simulink model "A13_17"  (R2017b)
settings: Solver=VariableStepAuto  StartTime=0.0  StopTime=20  RelTol=1e-3
settings Model: Creator=user  LastModifiedBy=user
settings SFSimCC: SimUseLocalCustomCode=on
settings RTWCC: RTWUseLocalCustomCode=on

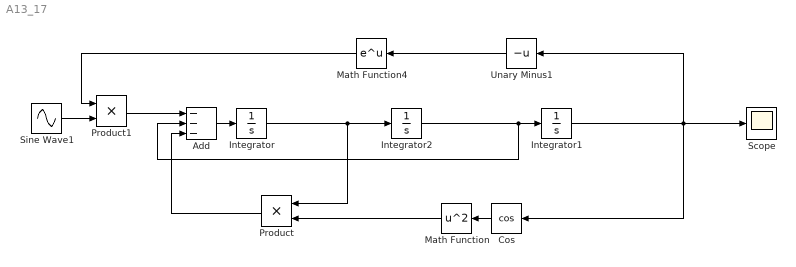
== system A13_17 ==
  Add : Sum  Inputs=---
  Cos : Trigonometry  Operator=cos
  Integrator : Integrator  InitialCondition=1
  Integrator1 : Integrator  InitialCondition=3
  Integrator2 : Integrator  InitialCondition=-2
  Math Function : Math  Operator=square  SaturateOnIntegerOverflow=on
  Math Function4 : Math  SaturateOnIntegerOverflow=on
  Product : Product
  Product1 : Product
  Scope : Scope
  Sine Wave1 : Sin  Frequency=10  SampleTime=0
  Unary Minus1 : UnaryMinus
  wires:
  Integrator/1 -> Integrator2/1, Product/1
  Integrator2/1 -> Add/2, Integrator1/1
  Integrator1/1 -> Unary Minus1/1, Cos/1, Scope/1
  Cos/1 -> Math Function/1
  Product/1 -> Add/3
  Add/1 -> Integrator/1
  Sine Wave1/1 -> Product1/2
  Math Function4/1 -> Product1/1
  Product1/1 -> Add/1
  Unary Minus1/1 -> Math Function4/1
  Math Function/1 -> Product/2
